simulink library "buoyEng_ul"  (R2020a)
settings: Solver=VariableStepAuto  StartTime=0.0  StopTime=10.0  RelTol=1e-3
values from neighbouring files (symbols this model uses):
  momentArm = [0 0 0]    [buoyEng_ts.m]
libraries: vrlib x1, eulAng2RotMat_ul x1
settings Model: Creator=mitch  LastModifiedBy=mitch

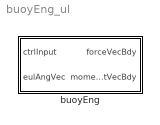
== system buoyEng_ul ==
  buoyEng : Subsystem

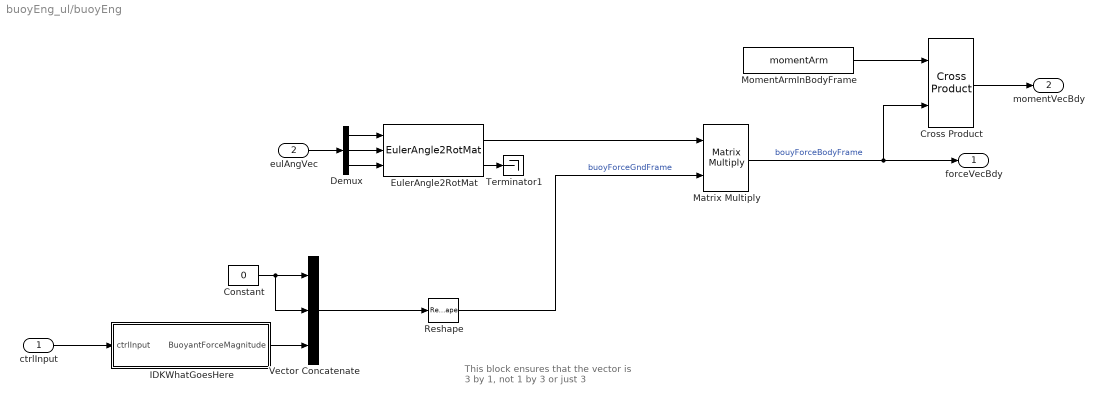
== system buoyEng_ul/buoyEng ==
  note: This block ensures that the
      | vector is 3 by 1, not 1 by 3 or just 3
  ctrlInput : Inport
  eulAngVec : Inport  Port=2
  Constant : Constant  Value=0
  Cross Product : vrlib/Utilities/Cross Product
  Demux : Demux  Outputs=3
  EulerAngle2RotMat : eulAng2RotMat_ul/EulerAngle2RotMat  SystemSampleTime=-1  Latency=0  AutoFrameSizeCalculation=off
  IDKWhatGoesHere : Subsystem
  Matrix Multiply : Product  Multiplication=Matrix(*)
  MomentArmInBodyFrame : Constant  Value=momentArm
  Reshape : Reshape  OutputDimensionality=Column vector (2-D)
  Terminator1 : Terminator
  Vector Concatenate : Concatenate  NumInputs=3
  forceVecBdy : Outport
  momentVecBdy : Outport  Port=2
  wires:
  eulAngVec/1 -> Demux/1
  EulerAngle2RotMat/2 -> Terminator1/1
  Matrix Multiply/1 -> Cross Product/2, forceVecBdy/1  "bouyForceBodyFrame"
  Demux/3 -> EulerAngle2RotMat/3
  Demux/1 -> EulerAngle2RotMat/1
  Demux/2 -> EulerAngle2RotMat/2
  ctrlInput/1 -> IDKWhatGoesHere/1(ctrlInput)
  IDKWhatGoesHere/1(BuoyantForceMagnitude) -> Vector Concatenate/3
  Constant/1 -> Vector Concatenate/2, Vector Concatenate/1
  Vector Concatenate/1 -> Reshape/1
  Reshape/1 -> Matrix Multiply/2  "buoyForceGndFrame"
  Cross Product/1 -> momentVecBdy/1
  MomentArmInBodyFrame/1 -> Cross Product/1
  EulerAngle2RotMat/1 -> Matrix Multiply/1

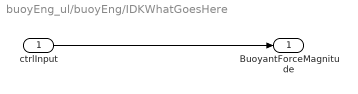
== system buoyEng_ul/buoyEng/IDKWhatGoesHere ==
  ctrlInput : Inport
  BuoyantForceMagnitude : Outport
  wires:
  ctrlInput/1 -> BuoyantForceMagnitude/1
